simulink model "Integration_Forward_JFK"  (R2015a)
settings: Solver=ode5  StartTime=0.0  StopTime=350  FixedStep=0.01  MaxStep=0.01  RelTol=1e-3
values from neighbouring files (symbols this model uses):
  H0 = interp1q(Periodic_Solution(:,1),Periodic_Solution(:,4),time_shift(n))    [Gradient_Descent_Controllable_Sleeping.m]
  Periodic_Solution = Periodic_Solution(Initial_Time*100+1:end,:)    [Gradient_Descent_Controllable_Sleeping.m]    (also in Periodic_Solution_JFK_u_1000lux.mat = [0 0.00999999999999 0.02 0.03 0.04 0.05 0.0599999999999 0.06)
  Sleep0 = 0    [Gradient_Descent_Controllable_Sleeping.m]
  Sleep_update = Sleep    [Gradient_Descent_Controllable_Sleeping.m]
  tol = 0.01    [Gradient_Descent_Controllable_Sleeping.m]
  u_update = u    [Gradient_Descent_Controllable_Sleeping.m]
  x0 = interp1q(Periodic_Solution(:,1),Periodic_Solution(:,2),time_shift(n))    [Gradient_Descent_Controllable_Sleeping.m]
  xc0 = interp1q(Periodic_Solution(:,1),Periodic_Solution(:,3),time_shift(n))    [Gradient_Descent_Controllable_Sleeping.m]
settings Model: Creator=wangf7  LastModifiedBy=Jiawei Yin
settings OptimizationCC: ExpressionDepthLimit=2147483647
settings DebuggingCC: AlgebraicLoopMsg=none  ArtificialAlgebraicLoopMsg=none  UnderspecifiedInitializationDetection=Classic  MergeDetectMultiDrivingBlocksExec=none  SolverPrmCheckMsg=warning  StateNameClashWarn=warning

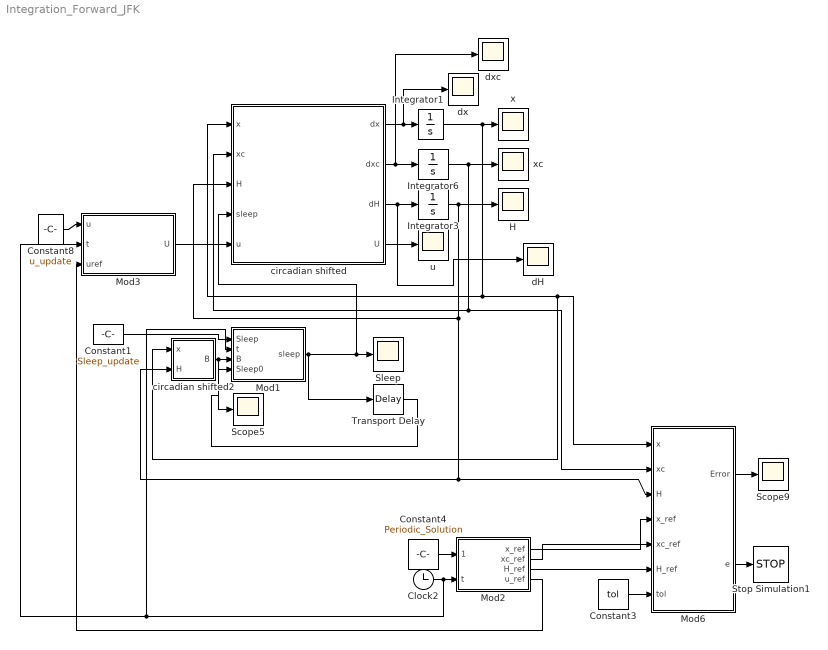
== system Integration_Forward_JFK ==
  Clock2 : Clock
  Constant1 : Constant  Value=Sleep_update
  Constant3 : Constant  Value=tol
  Constant4 : Constant  Value=Periodic_Solution
  Constant8 : Constant  Value=u_update
  H : Scope
      settings: TimeRange=auto  MaxDataPoints=5000  SaveName=H  YMin=-10  YMax=10  SampleTime=-1  DataFormat=Array
  Integrator1 : Integrator  InitialCondition=x0
  Integrator3 : Integrator  InitialCondition=H0
  Integrator6 : Integrator  InitialCondition=xc0
  Mod1 : MATLAB Function  TreatAsAtomicUnit=on
      settings: PermitHierarchicalResolution=ParametersOnly
  Mod2 : MATLAB Function  TreatAsAtomicUnit=on
      settings: PermitHierarchicalResolution=ParametersOnly
  Mod3 : MATLAB Function  TreatAsAtomicUnit=on
      settings: PermitHierarchicalResolution=ParametersOnly
  Mod6 : MATLAB Function  TreatAsAtomicUnit=on
      settings: PermitHierarchicalResolution=ParametersOnly
  Scope5 : Scope
      settings: TimeRange=auto  MaxDataPoints=5000  SaveName=B  YMin=-10  YMax=10  SampleTime=-1  DataFormat=Array
  Scope9 : Scope
      settings: TimeRange=auto  MaxDataPoints=5000  SaveName=Error  YMin=-10  YMax=10  SampleTime=-1  DataFormat=Array
  Sleep : Scope
      settings: TimeRange=auto  MaxDataPoints=5000  SaveName=Sleep  YMin=-10  YMax=10  SampleTime=-1  DataFormat=Array
  Stop Simulation1 : Stop
  Transport Delay : TransportDelay  DelayTime=.01  InitialOutput=Sleep0
  circadian shifted : MATLAB Function  TreatAsAtomicUnit=on
      settings: PermitHierarchicalResolution=ParametersOnly
  circadian shifted2 : MATLAB Function  TreatAsAtomicUnit=on
      settings: PermitHierarchicalResolution=ParametersOnly
  dH : Scope
      settings: TimeRange=auto  MaxDataPoints=5000  SaveName=dH  YMin=0.03966  YMax=0.05966  SampleTime=-1  DataFormat=Array
  dx : Scope
      settings: TimeRange=auto  MaxDataPoints=5000  SaveName=dx  YMin=-10  YMax=10  SampleTime=-1  DataFormat=Array
  dxc : Scope
      settings: TimeRange=auto  MaxDataPoints=5000  SaveName=dxc  YMin=-10  YMax=10  SampleTime=-1  DataFormat=Array
  u : Scope
      settings: TimeRange=auto  MaxDataPoints=5000  SaveName=u  YMin=-0.0276  YMax=0.2484  SampleTime=-1  DataFormat=Array
  x : Scope
      settings: TimeRange=auto  MaxDataPoints=5000  SaveName=x  YMin=-10  YMax=10  SampleTime=-1  DataFormat=Array
  xc : Scope
      settings: TimeRange=auto  MaxDataPoints=5000  SaveName=xc  YMin=-10  YMax=10  SampleTime=-1  DataFormat=Array
  wires:
  circadian shifted/1(dx) -> Integrator1/1, dx/1
  Integrator1/1 -> circadian shifted2/1(x), Mod6/1(x), circadian shifted/1(x), x/1
  Integrator6/1 -> Mod6/2(xc), circadian shifted/2(xc), xc/1
  circadian shifted2/1(B) -> Mod1/3(B), Scope5/1
  Mod1/1(sleep) -> Sleep/1, circadian shifted/4(sleep), Transport Delay/1
  Constant4/1 -> Mod2/1(Periodic_Solution)
  Mod6/2(e) -> Stop Simulation1/1
  Mod6/1(Error) -> Scope9/1
  Mod2/3(H_ref) -> Mod6/6(H_ref)
  Constant3/1 -> Mod6/7(tol)
  circadian shifted/2(dxc) -> Integrator6/1, dxc/1
  Integrator3/1 -> circadian shifted2/2(H), Mod6/3(H), circadian shifted/3(H), H/1
  Mod2/1(x_ref) -> Mod6/4(x_ref)
  Mod2/2(xc_ref) -> Mod6/5(xc_ref)
  Constant8/1 -> Mod3/1(u)
  Mod3/1(U) -> circadian shifted/5(u)
  circadian shifted/3(dH) -> dH/1, Integrator3/1
  circadian shifted/4(U) -> u/1
  Constant1/1 -> Mod1/1(Sleep)
  Clock2/1 -> Mod1/2(t), Mod3/2(t), Mod2/2(t)
  Transport Delay/1 -> Mod1/4(Sleep0)
  Mod2/4(u_ref) -> Mod3/3(uref)

== matlab function Integration_Forward_JFK/Mod1 ==
  data: Sleep input; sleep output; t input; B input; Sleep0 input
function sleep = fcn(Sleep,t,B,Sleep0)
%#codegen
if t<=Sleep(end,1)
    sleep=interp1q(Sleep(:,1),Sleep(:,2),t);
    if sleep==0 && Sleep0==1
        if B>0.27
            sleep=1;
        end
    elseif sleep==1 && Sleep0==0
        if B<0.67
            sleep=0;
        end
    end
    if B>0.77
        sleep=1;
    elseif B<0.17
        sleep=0;
    end
else
    sleep=Sleep0;
    if B>0.67
        sleep=1;
    elseif B<0.17
        sleep=0;
    end
end

== matlab function Integration_Forward_JFK/circadian shifted ==
  data: x input; xc input; H input; sleep input; u input; dx output; dxc output; dH output; U output
function [dx,dxc,dH,U] = fcn(x,xc,H,sleep,u)
%#eml

tr=18.2;
td=4.2;

q = 1/3;
taux = 24.2;
k = 0.55;
mu=0.13;
U= u*(1-sleep);
B = u*(1-0.4*x)*(1-0.4*xc)*(1-sleep);

dx = (pi/12)*(xc + B  + mu*(1/3*x + 4/3*x^3 - 256/105*x^7));
dxc = (pi/12)*(q*B *xc - (24/(taux*0.99729))^2*x - k*B*x);
dH = (1-sleep)*(1-H)/tr-(H*sleep)/td;

== matlab function Integration_Forward_JFK/circadian shifted2 ==
  data: x input; H input; B output
function B = fcn(x,H)
%#eml
B=H-0.1333*x;

== matlab function Integration_Forward_JFK/Mod2 ==
  data: Periodic_Solution input; x_ref output; xc_ref output; t input; H_ref output; u_ref output
function [x_ref,xc_ref,H_ref,u_ref] = fcn(Periodic_Solution,t)
%#codegen
x_ref=interp1q(Periodic_Solution(:,1),Periodic_Solution(:,2),t);
xc_ref=interp1q(Periodic_Solution(:,1),Periodic_Solution(:,3),t);
H_ref=interp1q(Periodic_Solution(:,1),Periodic_Solution(:,4),t);
%sleep_ref=interp1q(Periodic_Solution(:,1),Periodic_Solution(:,6),t);
u_ref=interp1q(Periodic_Solution(:,1),Periodic_Solution(:,5),t);

== matlab function Integration_Forward_JFK/Mod6 ==
  data: Error output; x input; xc input; H input; x_ref input; xc_ref input; e output; H_ref input; tol input
function [Error,e] = fcn(x,xc,H,x_ref,xc_ref,H_ref,tol)
%#codegen
Error=(H-H_ref)^2+(x-x_ref)^2+(xc-xc_ref)^2;
e=Error<tol;

== matlab function Integration_Forward_JFK/Mod3 ==
  data: u input; U output; t input; uref input
function U  = fcn(u,t,uref)
%#codegen
if t<=u(end,1)
    U=interp1q(u(:,1),u(:,2),t);
else
    U=uref;
end
